simulink model "QTIP1DOFSim"  (R2017a)
settings: Solver=ode3  StartTime=0.0  StopTime=10  FixedStep=0.001  RelTol=1e-3  EnableMultiTasking=on
settings Model: Creator=simose  LastModifiedBy=cjb3817
settings SolverCC: InitialStep=0.001
settings DataIOCC: LimitDataPoints=on  SaveFormat=Array
settings OptimizationCC: DefaultParameterBehavior=Inlined  BufferReuse=off  LifeSpan=inf
settings DebuggingCC: InitInArrayFormatMsg=none  SFUnexpectedBacktrackingDiag=warning  SFNoUnconditionalDefaultTransitionDiag=warning  SFExecutionAtInitializationDiag=none
settings HardwareCC: ProdBitPerPointer=32  ProdBitPerSizeT=32  ProdBitPerPtrDiffT=32  ProdLargestAtomicFloat=None  ProdIntDivRoundTo=Undefined  ProdEndianess=Unspecified  ProdWordSize=32  ProdHWDeviceType=32-bit Generic
settings ModelReferenceCC: PropagateSignalLabelsOutOfModel=off
settings GRTTargetCC: TargetLangStandard=C89/C90 (ANSI)  GeneratePreprocessorConditionals=Disable all
settings ConfigComp: CovMetricSettings=dw  CovHtmlReporting=on  CovSaveCumulativeToWorkspaceVar=on  CovSaveSingleToWorkspaceVar=on  CovExternalEMLEnable=off
settings SimscapeCC: SimscapeLogType=all  SimscapeLogDataHistory=10000
settings ConfigurationSet: Description=SimMechanics 2G

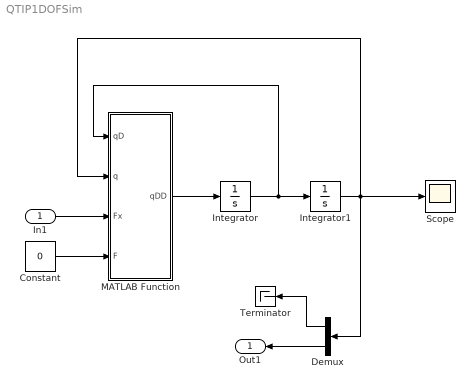
== system QTIP1DOFSim ==
  In1 : Inport
  Constant : Constant  Value=0
  Demux : Demux  Outputs=2
  Integrator : Integrator  InitialCondition=[0;0]
  Integrator1 : Integrator  InitialCondition=[0;0.1]
  MATLAB Function : MATLAB Function  TreatAsAtomicUnit=on
  Scope : Scope
  Terminator : Terminator
  Out1 : Outport
  wires:
  MATLAB Function/1(qDD) -> Integrator/1
  Integrator/1 -> Integrator1/1, MATLAB Function/1(qD)
  Integrator1/1 -> Scope/1, MATLAB Function/2(q), Demux/1
  Demux/1 -> Terminator/1
  In1/1 -> MATLAB Function/3(Fx)
  Demux/2 -> Out1/1
  Constant/1 -> MATLAB Function/4(F)

== matlab function QTIP1DOFSim/MATLAB Function ==
  data: qD input; q input; qDD output; Fx input; F input
function qDD = fcn(qD,q,Fx,F)

Mc = 1;
mp = 1;
J = 1;
d = 1.5;
l = 3;
g=9.81;

M = [Mc+mp, d*mp*cos(q(2)); d*mp*cos(q(2)), J+d^2*mp];
D = [0, -d*mp*sin(q(2))*qD(2); 0, 0];
G = [0; -d*g*mp*sin(q(2))];

T = [Fx-F*cos(q(2)); -F*l];

qDD = M\(T-D*qD-G);

end
